simulink model "uz_mpc_6ph"  (R2024b)
settings: Solver=FixedStepDiscrete  StartTime=0.0  StopTime=0.003  RelTol=1e-3
values from neighbouring files (symbols this model uses):
  IB = sqrt(2)*IR    [uz_mpc_6ph_init.m]    (also in uz_mpc_6ph_state_machine_init.m)
  id_ref = 0.0    (= 0)    [uz_mpc_6ph_init.m]    (also in uz_mpc_6ph_state_machine_init.m)
  iq_ref = 15.0    (= 15)    [uz_mpc_6ph_init.m]    (also in uz_mpc_6ph_state_machine_init.m = 3)
  ix_ref = 0.0    (= 0)    [uz_mpc_6ph_init.m]    (also in uz_mpc_6ph_state_machine_init.m)
  iy_ref = 0.0    (= 0)    [uz_mpc_6ph_init.m]    (also in uz_mpc_6ph_state_machine_init.m)
  lambda_d = 1.0    (= 1)    [uz_mpc_6ph_init.m]    (also in uz_mpc_6ph_state_machine_init.m)
  lambda_q = 1.0    (= 1)    [uz_mpc_6ph_init.m]    (also in uz_mpc_6ph_state_machine_init.m)
  lambda_u = 0.0    (= 0)    [uz_mpc_6ph_init.m]    (also in uz_mpc_6ph_state_machine_init.m)
  lambda_x = 1.0    (= 1)    [uz_mpc_6ph_init.m]    (also in uz_mpc_6ph_state_machine_init.m)
  lambda_y = 1.0    (= 1)    [uz_mpc_6ph_init.m]    (also in uz_mpc_6ph_state_machine_init.m)
  Ld_over_LB = Ld/LB    [uz_mpc_6ph_init.m]    (also in uz_mpc_6ph_state_machine_init.m)
  Lq_over_LB = Lq/LB    [uz_mpc_6ph_init.m]    (also in uz_mpc_6ph_state_machine_init.m)
  n_rpm = 2200.0    (= 2200)    [uz_mpc_6ph_init.m]    (also in uz_mpc_6ph_state_machine_init.m = 1200)
  omegaB = nR*2*pi()/60*p    [uz_mpc_6ph_init.m]    (also in uz_mpc_6ph_state_machine_init.m)
  p = 5    [uz_mpc_6ph_init.m]    (also in uz_mpc_6ph_state_machine_init.m)
  psi_pm_over_psiB = psi_pm/psiB    [uz_mpc_6ph_init.m]    (also in uz_mpc_6ph_state_machine_init.m)
  Rs_over_ZB = Rs/ZB    [uz_mpc_6ph_init.m]    (also in uz_mpc_6ph_state_machine_init.m)
  t_ADC = 1/f_ADC    (= 1e-05)    [uz_mpc_6ph_init.m]    (also in uz_mpc_6ph_state_machine_init.m)
  t_clock = 1/f_clock    (= 1e-08)    [uz_mpc_6ph_init.m]    (also in uz_mpc_6ph_state_machine_init.m)
  Ts_times_ZB_over_Ld = Ts*ZB/Ld    [uz_mpc_6ph_init.m]    (also in uz_mpc_6ph_state_machine_init.m)
  Ts_times_ZB_over_Lq = Ts*ZB/Lq    [uz_mpc_6ph_init.m]    (also in uz_mpc_6ph_state_machine_init.m)
  Ts_times_ZB_over_Lx = Ts*ZB/Lx    [uz_mpc_6ph_init.m]    (also in uz_mpc_6ph_state_machine_init.m)
  Ts_times_ZB_over_Ly = Ts*ZB/Ly    [uz_mpc_6ph_init.m]    (also in uz_mpc_6ph_state_machine_init.m)
  v_dc = 565.0    (= 565)    [uz_mpc_6ph_init.m]    (also in uz_mpc_6ph_state_machine_init.m)
  VB = sqrt(2/3)*VR    [uz_mpc_6ph_init.m]    (also in uz_mpc_6ph_state_machine_init.m)
libraries: nesl_utility x32, fl_lib x29, simulink x23, ee_lib x12, hdlsllib x2, spsAlphaBetaZerotodq0Lib x1, batteryecm_lib x1
(part 3 of 4)

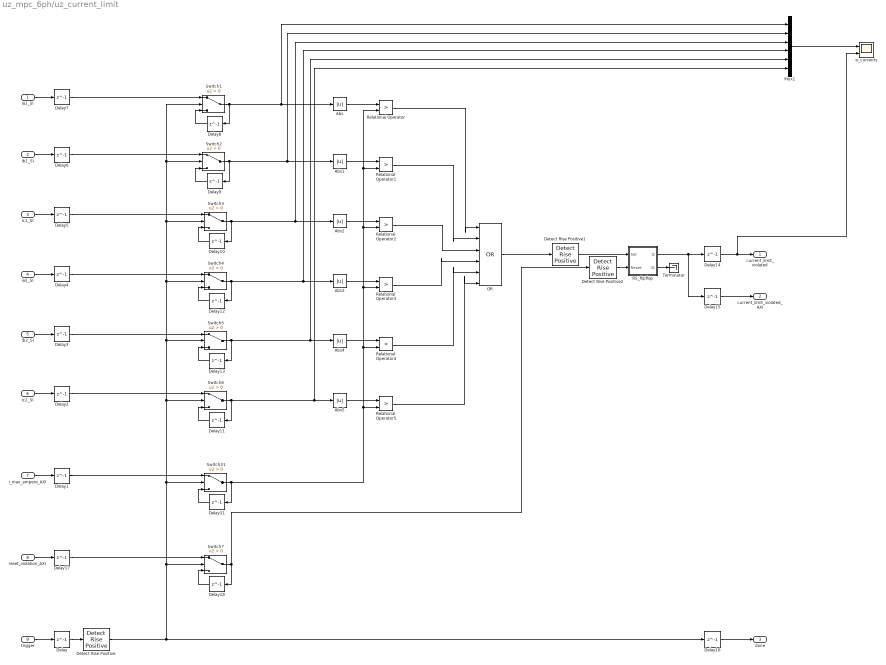
== system uz_mpc_6ph/uz_current_limit ==
  ia1_SI : Inport
  ib1_SI : Inport  Port=2
  ic1_SI : Inport  Port=3
  ia2_SI : Inport  Port=4
  ib2_SI : Inport  Port=5
  ic2_SI : Inport  Port=6
  i_max_ampere_AXI : Inport  Port=7
  reset_violation_AXI : Inport  Port=8
  trigger : Inport  Port=9
  Abs{,1..5} (6 alike) : Abs  SaturateOnIntegerOverflow=off
  Delay{,2..16} (16 alike) : Delay  DelayLength=1
  Delay{1,17..18,31} (4 alike) : Delay  DelayLength=1  InitialCondition=0
  Detect Rise Positive : simulink/Logic and Bit Operations/Detect Rise Positive  vinit=0  OutDataTypeStr=boolean
  Detect Rise Positive1 : simulink/Logic and Bit Operations/Detect Rise Positive  vinit=0  OutDataTypeStr=boolean
  Detect Rise Positive2 : simulink/Logic and Bit Operations/Detect Rise Positive  vinit=0  OutDataTypeStr=boolean
  Mux1 : Mux  Inputs=6
  OR : Logic  Operator=OR  Inputs=6  IconShape=distinctive  AllPortsSameDT=off  OutDataTypeStr=boolean
  RS_flipflop : Subsystem
  Relational Operator{,1..5} (6 alike) : RelationalOperator  Operator=>  OutDataTypeStr=boolean  RndMeth=Simplest  InputSameDT=off
  Switch{1..7,31} (8 alike) : Switch  Criteria=u2 > Threshold  SaturateOnIntegerOverflow=off  InputSameDT=off
  Terminator : Terminator
  si_currents : Scope  NumInputPorts=2
  current_limit_violated : Outport  VectorParamsAs1DForOutWhenUnconnected=off
  current_limit_violated_AXI : Outport  Port=2  VectorParamsAs1DForOutWhenUnconnected=off
  done : Outport  Port=3  VectorParamsAs1DForOutWhenUnconnected=off
  wires:
  Abs/1 -> Relational Operator/1
  Abs1/1 -> Relational Operator1/1
  Abs2/1 -> Relational Operator2/1
  Abs3/1 -> Relational Operator3/1
  Abs4/1 -> Relational Operator4/1
  Abs5/1 -> Relational Operator5/1
  Switch31/1 -> Relational Operator5/2, Relational Operator4/2, Relational Operator3/2, Relational Operator2/2, Relational Operator1/2, Relational Operator/2, Delay31/1
  trigger/1 -> Delay/1
  Delay/1 -> Detect Rise Positive/1
  Delay31/1 -> Switch31/3
  i_max_ampere_AXI/1 -> Delay1/1
  Delay1/1 -> Switch31/1
  ia1_SI/1 -> Delay7/1
  ib1_SI/1 -> Delay6/1
  ic1_SI/1 -> Delay5/1
  ia2_SI/1 -> Delay4/1
  ib2_SI/1 -> Delay3/1
  ic2_SI/1 -> Delay2/1
  Delay7/1 -> Switch1/1
  Delay6/1 -> Switch2/1
  Delay5/1 -> Switch3/1
  Delay4/1 -> Switch4/1
  Delay3/1 -> Switch5/1
  Delay2/1 -> Switch6/1
  Detect Rise Positive/1 -> Switch7/2, Switch6/2, Switch5/2, Switch4/2, Switch3/2, Switch2/2, Switch1/2, Switch31/2, Delay16/1
  Delay11/1 -> Switch6/3
  Delay13/1 -> Switch5/3
  Delay12/1 -> Switch4/3
  Delay10/1 -> Switch3/3
  Delay9/1 -> Switch2/3
  Delay8/1 -> Switch1/3
  Switch1/1 -> Mux1/1, Abs/1, Delay8/1
  Switch2/1 -> Delay9/1, Mux1/2, Abs1/1
  Switch3/1 -> Delay10/1, Mux1/3, Abs2/1
  Switch4/1 -> Delay12/1, Mux1/4, Abs3/1
  Switch5/1 -> Delay13/1, Mux1/5, Abs4/1
  Switch6/1 -> Delay11/1, Mux1/6, Abs5/1
  Relational Operator/1 -> OR/1
  Relational Operator1/1 -> OR/2
  Relational Operator2/1 -> OR/3
  Relational Operator3/1 -> OR/4
  Relational Operator5/1 -> OR/6
  OR/1 -> Detect Rise Positive1/1
  Delay16/1 -> done/1
  Delay15/1 -> current_limit_violated_AXI/1
  Relational Operator4/1 -> OR/5
  Mux1/1 -> si_currents/1
  Delay14/1 -> si_currents/2, current_limit_violated/1
  RS_flipflop/1(Q) -> Delay15/1, Delay14/1
  RS_flipflop/2(!Q) -> Terminator/1
  reset_violation_AXI/1 -> Delay17/1
  Delay18/1 -> Switch7/3
  Switch7/1 -> Delay18/1, Detect Rise Positive2/1
  Delay17/1 -> Switch7/1
  Detect Rise Positive1/1 -> RS_flipflop/1(Set)
  Detect Rise Positive2/1 -> RS_flipflop/2(Reset)

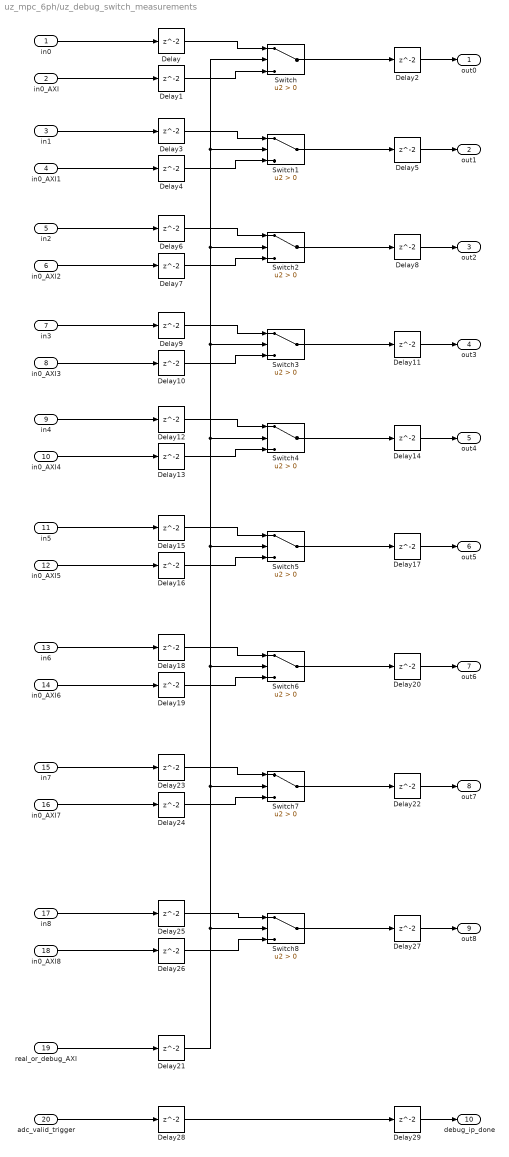
== system uz_mpc_6ph/uz_debug_switch_measurements ==
  in0 : Inport
  in0_AXI : Inport  Port=2
  in1 : Inport  Port=3
  in0_AXI1 : Inport  Port=4
  in2 : Inport  Port=5
  in0_AXI2 : Inport  Port=6
  in3 : Inport  Port=7
  in0_AXI3 : Inport  Port=8
  in4 : Inport  Port=9
  in0_AXI4 : Inport  Port=10
  in5 : Inport  Port=11
  in0_AXI5 : Inport  Port=12
  in6 : Inport  Port=13
  in0_AXI6 : Inport  Port=14
  in7 : Inport  Port=15
  in0_AXI7 : Inport  Port=16
  in8 : Inport  Port=17
  in0_AXI8 : Inport  Port=18
  real_or_debug_AXI : Inport  Port=19
  adc_valid_trigger : Inport  Port=20
  Delay{,1..29} (30 alike) : Delay
  Switch{,1..8} (9 alike) : Switch  Criteria=u2 > Threshold  SaturateOnIntegerOverflow=off  InputSameDT=off
  out0 : Outport  VectorParamsAs1DForOutWhenUnconnected=off
  out1 : Outport  Port=2  VectorParamsAs1DForOutWhenUnconnected=off
  out2 : Outport  Port=3  VectorParamsAs1DForOutWhenUnconnected=off
  out3 : Outport  Port=4  VectorParamsAs1DForOutWhenUnconnected=off
  out4 : Outport  Port=5  VectorParamsAs1DForOutWhenUnconnected=off
  out5 : Outport  Port=6  VectorParamsAs1DForOutWhenUnconnected=off
  out6 : Outport  Port=7  VectorParamsAs1DForOutWhenUnconnected=off
  out7 : Outport  Port=8  VectorParamsAs1DForOutWhenUnconnected=off
  out8 : Outport  Port=9  VectorParamsAs1DForOutWhenUnconnected=off
  debug_ip_done : Outport  Port=10  VectorParamsAs1DForOutWhenUnconnected=off
  wires:
  in0/1 -> Delay/1
  in0_AXI/1 -> Delay1/1
  Delay/1 -> Switch/1
  Delay1/1 -> Switch/3
  Switch/1 -> Delay2/1
  Delay2/1 -> out0/1
  in0_AXI1/1 -> Delay4/1
  Delay5/1 -> out1/1
  in1/1 -> Delay3/1
  Delay4/1 -> Switch1/3
  Delay3/1 -> Switch1/1
  Switch1/1 -> Delay5/1
  in0_AXI2/1 -> Delay7/1
  Delay8/1 -> out2/1
  in2/1 -> Delay6/1
  Delay7/1 -> Switch2/3
  Delay6/1 -> Switch2/1
  Switch2/1 -> Delay8/1
  in0_AXI3/1 -> Delay10/1
  Delay11/1 -> out3/1
  in3/1 -> Delay9/1
  Delay10/1 -> Switch3/3
  Delay9/1 -> Switch3/1
  Switch3/1 -> Delay11/1
  in0_AXI4/1 -> Delay13/1
  Delay14/1 -> out4/1
  in4/1 -> Delay12/1
  Delay13/1 -> Switch4/3
  Delay12/1 -> Switch4/1
  Switch4/1 -> Delay14/1
  in0_AXI5/1 -> Delay16/1
  Delay17/1 -> out5/1
  in5/1 -> Delay15/1
  Delay16/1 -> Switch5/3
  Delay15/1 -> Switch5/1
  Switch5/1 -> Delay17/1
  in0_AXI6/1 -> Delay19/1
  Delay20/1 -> out6/1
  in6/1 -> Delay18/1
  Delay19/1 -> Switch6/3
  Delay18/1 -> Switch6/1
  Switch6/1 -> Delay20/1
  real_or_debug_AXI/1 -> Delay21/1
  Delay22/1 -> out7/1
  Delay23/1 -> Switch7/1
  Delay24/1 -> Switch7/3
  Switch7/1 -> Delay22/1
  in0_AXI7/1 -> Delay24/1
  in7/1 -> Delay23/1
  in0_AXI8/1 -> Delay26/1
  in8/1 -> Delay25/1
  Delay27/1 -> out8/1
  Switch8/1 -> Delay27/1
  Delay25/1 -> Switch8/1
  Delay26/1 -> Switch8/3
  Delay21/1 -> Switch/2, Switch1/2, Switch2/2, Switch3/2, Switch4/2, Switch5/2, Switch6/2, Switch7/2, Switch8/2
  Delay28/1 -> Delay29/1
  Delay29/1 -> debug_ip_done/1
  adc_valid_trigger/1 -> Delay28/1

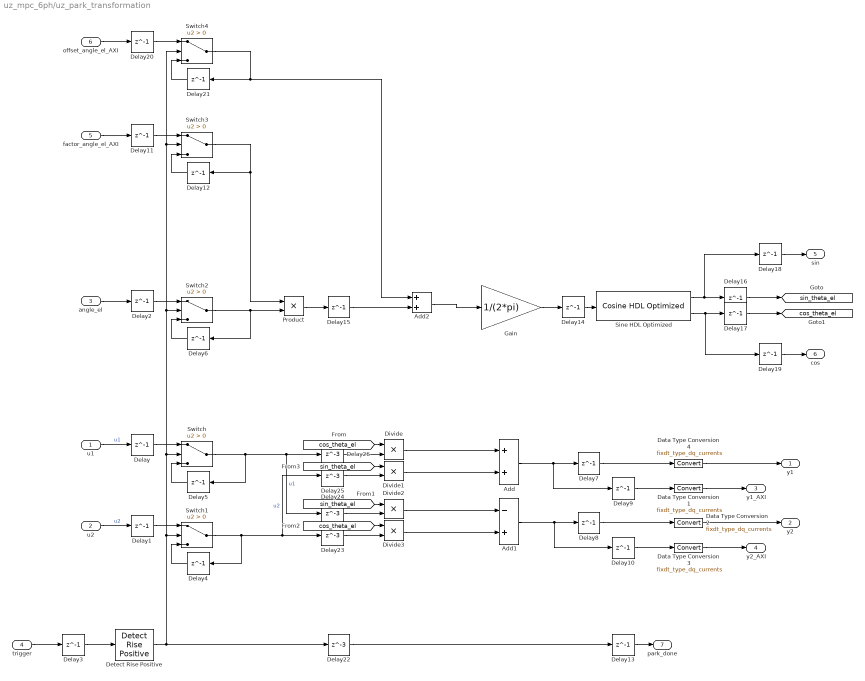
== system uz_mpc_6ph/uz_park_transformation ==
  u1 : Inport
  u2 : Inport  Port=2
  angle_el : Inport  Port=3
  trigger : Inport  Port=4
  factor_angle_el_AXI : Inport  Port=5
  offset_angle_el_AXI : Inport  Port=6
  Add : Sum  OutDataTypeStr=fixdt(1,27,16)
  Add1 : Sum  Inputs=-+  OutDataTypeStr=fixdt(1,27,16)
  Add2 : Sum  AccumDataTypeStr=fixdt(1,27,20)
  Data Type Conversion{1..4} (4 alike) : DataTypeConversion  OutDataTypeStr=fixdt_type_dq_currents  SaturateOnIntegerOverflow=off  RndMeth=Floor
  Delay{,1..21} (22 alike) : Delay  DelayLength=1
  Delay{22..26} (5 alike) : Delay  DelayLength=3
  Detect Rise Positive : simulink/Logic and Bit Operations/Detect Rise Positive  vinit=0  OutDataTypeStr=boolean
  Divide{,1..3} (4 alike) : Product  Inputs=**  OutDataTypeStr=fixdt(1,27,16)
  Gain : Gain  Gain=1/(2*pi)  OutDataTypeStr=fixdt(1,27,20)
  Product : Product  OutDataTypeStr=fixdt(1,27,20)
  Sine HDL Optimized : hdlsllib/Lookup Tables/Cosine HDL Optimized  OutputFormula=sin(2*pi*u) and cos(2*pi*u)  NumDataPoints=256  TableDataTypeStr=fixdt(0,26,20)  SimulateLUTROMDelay=off
  Switch{,1..4} (5 alike) : Switch  Criteria=u2 > Threshold  SaturateOnIntegerOverflow=off  InputSameDT=off
  y1 : Outport  VectorParamsAs1DForOutWhenUnconnected=off
  y2 : Outport  Port=2  VectorParamsAs1DForOutWhenUnconnected=off
  y1_AXI : Outport  Port=3  VectorParamsAs1DForOutWhenUnconnected=off
  y2_AXI : Outport  Port=4  VectorParamsAs1DForOutWhenUnconnected=off
  sin : Outport  Port=5  VectorParamsAs1DForOutWhenUnconnected=off
  cos : Outport  Port=6  VectorParamsAs1DForOutWhenUnconnected=off
  park_done : Outport  Port=7  VectorParamsAs1DForOutWhenUnconnected=off
  tag scope: cos_theta_el=global, sin_theta_el=global
  wires:
  Switch1/1 -> Delay4/1, Delay25/1, Delay23/1  "u2"
  Divide2/1 -> Add1/1
  Divide3/1 -> Add1/2
  [cos_theta_el] -> Divide3/1
  Switch/1 -> Delay24/1, Delay26/1, Delay5/1  "u1"
  [sin_theta_el] -> Divide2/1
  Divide1/1 -> Add/2
  [cos_theta_el] -> Divide/1
  [sin_theta_el] -> Divide1/1
  Add/1 -> Delay9/1, Delay7/1
  Add1/1 -> Delay10/1, Delay8/1
  Divide/1 -> Add/1
  angle_el/1 -> Delay2/1
  Sine HDL Optimized/2 -> Delay19/1, Delay17/1
  Sine HDL Optimized/1 -> Delay18/1, Delay16/1
  Gain/1 -> Delay14/1
  u1/1 -> Delay/1  "u1"
  u2/1 -> Delay1/1  "u2"
  Delay/1 -> Switch/1
  Delay1/1 -> Switch1/1
  Delay2/1 -> Switch2/1
  trigger/1 -> Delay3/1
  Delay4/1 -> Switch1/3
  Delay5/1 -> Switch/3
  Delay6/1 -> Switch2/3
  Delay7/1 -> Data Type Conversion4/1
  Switch2/1 -> Product/2, Delay6/1
  Switch3/1 -> Product/1, Delay12/1
  factor_angle_el_AXI/1 -> Delay11/1
  Delay12/1 -> Switch3/3
  Delay11/1 -> Switch3/1
  Product/1 -> Delay15/1
  Delay3/1 -> Detect Rise Positive/1
  Delay13/1 -> park_done/1
  Delay14/1 -> Sine HDL Optimized/1
  Delay16/1 -> [sin_theta_el]
  Delay17/1 -> [cos_theta_el]
  Delay18/1 -> sin/1
  Delay19/1 -> cos/1
  Add2/1 -> Gain/1
  Delay20/1 -> Switch4/1
  Switch4/1 -> Add2/1, Delay21/1
  Detect Rise Positive/1 -> Delay22/1, Switch1/2, Switch/2, Switch4/2, Switch3/2, Switch2/2
  Delay21/1 -> Switch4/3
  offset_angle_el_AXI/1 -> Delay20/1
  Delay15/1 -> Add2/2
  Delay22/1 -> Delay13/1
  Delay23/1 -> Divide3/2
  Delay24/1 -> Divide2/2
  Delay25/1 -> Divide1/2
  Delay26/1 -> Divide/2
  Data Type Conversion4/1 -> y1/1
  Delay9/1 -> Data Type Conversion1/1
  Delay8/1 -> Data Type Conversion2/1
  Delay10/1 -> Data Type Conversion3/1
  Data Type Conversion1/1 -> y1_AXI/1
  Data Type Conversion2/1 -> y2/1
  Data Type Conversion3/1 -> y2_AXI/1

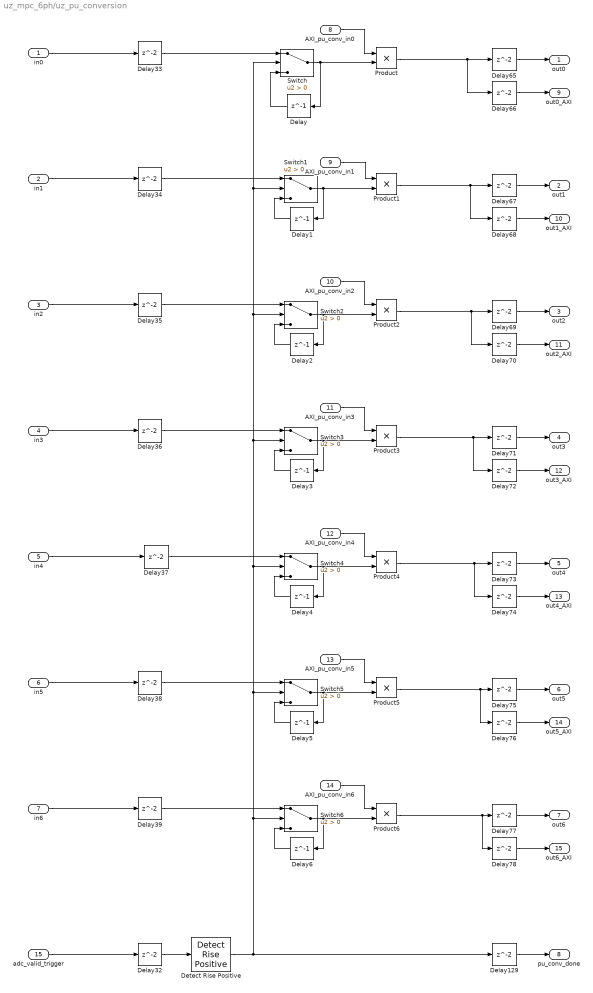
== system uz_mpc_6ph/uz_pu_conversion ==
  in0 : Inport  OutDataTypeStr=fixdt(1,27,15)
  in1 : Inport  Port=2  OutDataTypeStr=fixdt(1,27,15)
  in2 : Inport  Port=3  OutDataTypeStr=fixdt(1,27,15)
  in3 : Inport  Port=4  OutDataTypeStr=fixdt(1,27,15)
  in4 : Inport  Port=5  OutDataTypeStr=fixdt(1,27,15)
  in5 : Inport  Port=6  OutDataTypeStr=fixdt(1,27,15)
  in6 : Inport  Port=7  OutDataTypeStr=fixdt(1,27,15)
  AXI_pu_conv_in0 : Inport  Port=8  OutDataTypeStr=fixdt(0,18,18)
  AXI_pu_conv_in1 : Inport  Port=9  OutDataTypeStr=fixdt(0,18,18)
  AXI_pu_conv_in2 : Inport  Port=10  OutDataTypeStr=fixdt(0,18,18)
  AXI_pu_conv_in3 : Inport  Port=11  OutDataTypeStr=fixdt(0,18,18)
  AXI_pu_conv_in4 : Inport  Port=12  OutDataTypeStr=fixdt(0,18,18)
  AXI_pu_conv_in5 : Inport  Port=13  OutDataTypeStr=fixdt(0,18,18)
  AXI_pu_conv_in6 : Inport  Port=14  OutDataTypeStr=fixdt(0,18,18)
  adc_valid_trigger : Inport  Port=15  OutDataTypeStr=boolean
  Delay{,1..6} (7 alike) : Delay  DelayLength=1
  Delay{32..39,65..78,129} (23 alike) : Delay
  Detect Rise Positive : simulink/Logic and Bit Operations/Detect Rise Positive  vinit=0  OutDataTypeStr=boolean
  Product{,1..6} (7 alike) : Product  OutDataTypeStr=pu_fixdt_type
  Switch{,1..6} (7 alike) : Switch  Criteria=u2 > Threshold  SaturateOnIntegerOverflow=off  InputSameDT=off
  out0 : Outport
  out1 : Outport  Port=2
  out2 : Outport  Port=3
  out3 : Outport  Port=4
  out4 : Outport  Port=5
  out5 : Outport  Port=6
  out6 : Outport  Port=7
  pu_conv_done : Outport  Port=8  OutDataTypeStr=boolean  LockScale=on
  out0_AXI : Outport  Port=9
  out1_AXI : Outport  Port=10
  out2_AXI : Outport  Port=11
  out3_AXI : Outport  Port=12
  out4_AXI : Outport  Port=13
  out5_AXI : Outport  Port=14
  out6_AXI : Outport  Port=15
  wires:
  AXI_pu_conv_in0/1 -> Product/1
  Product/1 -> Delay65/1, Delay66/1
  AXI_pu_conv_in1/1 -> Product1/1
  Product1/1 -> Delay67/1, Delay68/1
  AXI_pu_conv_in2/1 -> Product2/1
  Product3/1 -> Delay71/1, Delay72/1
  Product2/1 -> Delay69/1, Delay70/1
  AXI_pu_conv_in3/1 -> Product3/1
  AXI_pu_conv_in4/1 -> Product4/1
  Product6/1 -> Delay77/1, Delay78/1
  Product5/1 -> Delay75/1, Delay76/1
  AXI_pu_conv_in6/1 -> Product6/1
  Product4/1 -> Delay73/1, Delay74/1
  AXI_pu_conv_in5/1 -> Product5/1
  Switch/1 -> Product/2, Delay/1
  Delay/1 -> Switch/3
  Switch1/1 -> Product1/2, Delay1/1
  Delay1/1 -> Switch1/3
  Switch2/1 -> Product2/2, Delay2/1
  Delay2/1 -> Switch2/3
  Switch3/1 -> Product3/2, Delay3/1
  Delay3/1 -> Switch3/3
  Switch4/1 -> Product4/2, Delay4/1
  Delay4/1 -> Switch4/3
  Switch5/1 -> Product5/2, Delay5/1
  Delay5/1 -> Switch5/3
  Switch6/1 -> Product6/2, Delay6/1
  Delay6/1 -> Switch6/3
  Detect Rise Positive/1 -> Delay129/1, Switch6/2, Switch5/2, Switch3/2, Switch2/2, Switch1/2, Switch/2, Switch4/2
  adc_valid_trigger/1 -> Delay32/1
  Delay32/1 -> Detect Rise Positive/1
  in0/1 -> Delay33/1
  Delay33/1 -> Switch/1
  in1/1 -> Delay34/1
  Delay34/1 -> Switch1/1
  in2/1 -> Delay35/1
  Delay35/1 -> Switch2/1
  in3/1 -> Delay36/1
  Delay36/1 -> Switch3/1
  in4/1 -> Delay37/1
  Delay37/1 -> Switch4/1
  in5/1 -> Delay38/1
  Delay38/1 -> Switch5/1
  in6/1 -> Delay39/1
  Delay39/1 -> Switch6/1
  Delay65/1 -> out0/1
  Delay66/1 -> out0_AXI/1
  Delay67/1 -> out1/1
  Delay68/1 -> out1_AXI/1
  Delay69/1 -> out2/1
  Delay70/1 -> out2_AXI/1
  Delay71/1 -> out3/1
  Delay72/1 -> out3_AXI/1
  Delay73/1 -> out4/1
  Delay74/1 -> out4_AXI/1
  Delay75/1 -> out5/1
  Delay76/1 -> out5_AXI/1
  Delay77/1 -> out6/1
  Delay78/1 -> out6_AXI/1
  Delay129/1 -> pu_conv_done/1

== system uz_mpc_6ph/uz_vsd_6ph_30deg ==
  a1 : Inport
  b1 : Inport  Port=2
  c1 : Inport  Port=3
  a2 : Inport  Port=4
  b2 : Inport  Port=5
  c2 : Inport  Port=6
  pu_conv_valid : Inport  Port=7
  Delay{,1..5} (6 alike) : Delay  DelayLength=1
  Delay{6..25} (20 alike) : Delay
  Detect Rise Positive : simulink/Logic and Bit Operations/Detect Rise Positive  vinit=0  OutDataTypeStr=boolean
  Switch{,1..5} (6 alike) : Switch  Criteria=u2 > Threshold  OutDataTypeStr=fixdt_type_vsd  SaturateOnIntegerOverflow=off  InputSameDT=off
  VSD_6ph_30deg : MATLAB Function  TreatAsAtomicUnit=on
  alpha : Outport  OutDataTypeStr=fixdt(1,18,11)  VectorParamsAs1DForOutWhenUnconnected=off
  beta : Outport  Port=2  OutDataTypeStr=fixdt(1,18,11)  VectorParamsAs1DForOutWhenUnconnected=off
  x1 : Outport  Port=3  OutDataTypeStr=fixdt(1,18,11)  VectorParamsAs1DForOutWhenUnconnected=off
  y1 : Outport  Port=4  OutDataTypeStr=fixdt(1,18,11)  VectorParamsAs1DForOutWhenUnconnected=off
  z1 : Outport  Port=5  OutDataTypeStr=fixdt(1,18,11)  VectorParamsAs1DForOutWhenUnconnected=off
  z2 : Outport  Port=6  OutDataTypeStr=fixdt(1,18,11)  VectorParamsAs1DForOutWhenUnconnected=off
  vsd_done : Outport  Port=7  VectorParamsAs1DForOutWhenUnconnected=off
  alpha_AXI : Outport  Port=8  OutDataTypeStr=fixdt(1,18,11)  VectorParamsAs1DForOutWhenUnconnected=off
  beta_AXI : Outport  Port=9  OutDataTypeStr=fixdt(1,18,11)  VectorParamsAs1DForOutWhenUnconnected=off
  x_AXI : Outport  Port=10  OutDataTypeStr=fixdt(1,18,11)  VectorParamsAs1DForOutWhenUnconnected=off
  y_AXI : Outport  Port=11  OutDataTypeStr=fixdt(1,18,11)  VectorParamsAs1DForOutWhenUnconnected=off
  z1_AXI : Outport  Port=12  OutDataTypeStr=fixdt(1,18,11)  VectorParamsAs1DForOutWhenUnconnected=off
  z2_AXI : Outport  Port=13  OutDataTypeStr=fixdt(1,18,11)  VectorParamsAs1DForOutWhenUnconnected=off
  wires:
  VSD_6ph_30deg/1(alpha) -> Delay20/1, Delay14/1
  VSD_6ph_30deg/2(beta) -> Delay21/1, Delay15/1
  VSD_6ph_30deg/3(x1) -> Delay22/1, Delay16/1
  VSD_6ph_30deg/4(y1) -> Delay23/1, Delay17/1
  VSD_6ph_30deg/5(z1) -> Delay24/1, Delay18/1
  VSD_6ph_30deg/6(z2) -> Delay25/1, Delay19/1
  pu_conv_valid/1 -> Delay6/1
  Detect Rise Positive/1 -> Switch5/2, Switch4/2, Switch3/2, Switch2/2, Switch1/2, Switch/2, Delay13/1
  Delay/1 -> Switch/3
  Switch/1 -> VSD_6ph_30deg/1(a1), Delay/1
  Delay1/1 -> Switch1/3
  Switch1/1 -> VSD_6ph_30deg/2(b1), Delay1/1
  Delay2/1 -> Switch2/3
  Switch2/1 -> VSD_6ph_30deg/3(c1), Delay2/1
  Delay3/1 -> Switch3/3
  Switch3/1 -> VSD_6ph_30deg/4(a2), Delay3/1
  Delay4/1 -> Switch4/3
  Switch4/1 -> VSD_6ph_30deg/5(b2), Delay4/1
  Delay5/1 -> Switch5/3
  Switch5/1 -> VSD_6ph_30deg/6(c2), Delay5/1
  a1/1 -> Delay7/1
  b1/1 -> Delay8/1
  c1/1 -> Delay9/1
  a2/1 -> Delay10/1
  b2/1 -> Delay11/1
  c2/1 -> Delay12/1
  Delay6/1 -> Detect Rise Positive/1
  Delay7/1 -> Switch/1
  Delay8/1 -> Switch1/1
  Delay9/1 -> Switch2/1
  Delay10/1 -> Switch3/1
  Delay11/1 -> Switch4/1
  Delay12/1 -> Switch5/1
  Delay13/1 -> vsd_done/1
  Delay14/1 -> alpha/1
  Delay15/1 -> beta/1
  Delay16/1 -> x1/1
  Delay17/1 -> y1/1
  Delay18/1 -> z1/1
  Delay19/1 -> z2/1
  Delay20/1 -> alpha_AXI/1
  Delay21/1 -> beta_AXI/1
  Delay22/1 -> x_AXI/1
  Delay23/1 -> y_AXI/1
  Delay24/1 -> z1_AXI/1
  Delay25/1 -> z2_AXI/1

== system uz_mpc_6ph/ctrl_state_machine/Subsystem ==
  Set : Inport
  Reset : Inport  Port=2
  Constant1 : Constant  Value=0  OutDataTypeStr=uint32  SampleTime=-1
  Data Type Conversion1 : DataTypeConversion  OutDataTypeStr=boolean  SaturateOnIntegerOverflow=off  RndMeth=Floor
  Data Type Conversion2 : DataTypeConversion  OutDataTypeStr=boolean  SaturateOnIntegerOverflow=off  RndMeth=Floor
  Logical Operator : Logic  Operator=NOT  AllPortsSameDT=off  OutDataTypeStr=boolean
  Logical Operator1 : Logic  AllPortsSameDT=off  OutDataTypeStr=boolean
  Logical Operator2 : Logic  Operator=OR  AllPortsSameDT=off  OutDataTypeStr=boolean
  Logical Operator3 : Logic  Operator=NOT  AllPortsSameDT=off  OutDataTypeStr=boolean
  Logical Operator4 : Logic  Operator=OR  AllPortsSameDT=off  OutDataTypeStr=boolean
  Logical Operator5 : Logic  AllPortsSameDT=off  OutDataTypeStr=boolean
  Switch1 : Switch  Criteria=u2 > Threshold  Threshold=1  SaturateOnIntegerOverflow=off  InputSameDT=off
  Unit Delay : UnitDelay  InitialCondition=1  SampleTime=t_clock  HasFrameUpgradeWarning=on
  Q : Outport  VectorParamsAs1DForOutWhenUnconnected=off
  !Q : Outport  Port=2  VectorParamsAs1DForOutWhenUnconnected=off
  wires:
  Logical Operator/1 -> Logical Operator1/2, Logical Operator5/1
  Reset/1 -> Data Type Conversion2/1
  Constant1/1 -> Switch1/2
  Logical Operator4/1 -> Switch1/1
  Data Type Conversion1/1 -> Logical Operator2/1, Logical Operator4/1
  Switch1/1 -> Q/1, Unit Delay/1, Logical Operator3/1
  Logical Operator3/1 -> !Q/1
  Set/1 -> Data Type Conversion1/1
  Logical Operator2/1 -> Logical Operator1/1
  Unit Delay/1 -> Logical Operator2/2, Logical Operator5/2
  Logical Operator5/1 -> Logical Operator4/2
  Logical Operator1/1 -> Switch1/3
  Data Type Conversion2/1 -> Logical Operator/1

== system uz_mpc_6ph/ctrl_state_machine/Subsystem2 ==
  Set : Inport
  Reset : Inport  Port=2
  Constant1 : Constant  Value=0  OutDataTypeStr=uint32  SampleTime=-1
  Data Type Conversion1 : DataTypeConversion  OutDataTypeStr=boolean  SaturateOnIntegerOverflow=off  RndMeth=Floor
  Data Type Conversion2 : DataTypeConversion  OutDataTypeStr=boolean  SaturateOnIntegerOverflow=off  RndMeth=Floor
  Logical Operator : Logic  Operator=NOT  AllPortsSameDT=off  OutDataTypeStr=boolean
  Logical Operator1 : Logic  AllPortsSameDT=off  OutDataTypeStr=boolean
  Logical Operator2 : Logic  Operator=OR  AllPortsSameDT=off  OutDataTypeStr=boolean
  Logical Operator3 : Logic  Operator=NOT  AllPortsSameDT=off  OutDataTypeStr=boolean
  Logical Operator4 : Logic  Operator=OR  AllPortsSameDT=off  OutDataTypeStr=boolean
  Logical Operator5 : Logic  AllPortsSameDT=off  OutDataTypeStr=boolean
  Switch1 : Switch  Criteria=u2 > Threshold  Threshold=1  SaturateOnIntegerOverflow=off  InputSameDT=off
  Unit Delay : UnitDelay  SampleTime=t_clock  HasFrameUpgradeWarning=on
  Q : Outport  VectorParamsAs1DForOutWhenUnconnected=off
  !Q : Outport  Port=2  VectorParamsAs1DForOutWhenUnconnected=off
  wires:
  Logical Operator/1 -> Logical Operator1/2, Logical Operator5/1
  Reset/1 -> Data Type Conversion2/1
  Constant1/1 -> Switch1/2
  Logical Operator4/1 -> Switch1/1
  Data Type Conversion1/1 -> Logical Operator2/1, Logical Operator4/1
  Switch1/1 -> Q/1, Unit Delay/1, Logical Operator3/1
  Logical Operator3/1 -> !Q/1
  Set/1 -> Data Type Conversion1/1
  Logical Operator2/1 -> Logical Operator1/1
  Unit Delay/1 -> Logical Operator2/2, Logical Operator5/2
  Logical Operator5/1 -> Logical Operator4/2
  Logical Operator1/1 -> Switch1/3
  Data Type Conversion2/1 -> Logical Operator/1

== system uz_mpc_6ph/ctrl_state_machine/Subsystem4 ==
  Set : Inport
  Reset : Inport  Port=2
  Constant1 : Constant  Value=0  OutDataTypeStr=uint32  SampleTime=-1
  Data Type Conversion1 : DataTypeConversion  OutDataTypeStr=boolean  SaturateOnIntegerOverflow=off  RndMeth=Floor
  Data Type Conversion2 : DataTypeConversion  OutDataTypeStr=boolean  SaturateOnIntegerOverflow=off  RndMeth=Floor
  Logical Operator : Logic  Operator=NOT  AllPortsSameDT=off  OutDataTypeStr=boolean
  Logical Operator1 : Logic  AllPortsSameDT=off  OutDataTypeStr=boolean
  Logical Operator2 : Logic  Operator=OR  AllPortsSameDT=off  OutDataTypeStr=boolean
  Logical Operator3 : Logic  Operator=NOT  AllPortsSameDT=off  OutDataTypeStr=boolean
  Logical Operator4 : Logic  Operator=OR  AllPortsSameDT=off  OutDataTypeStr=boolean
  Logical Operator5 : Logic  AllPortsSameDT=off  OutDataTypeStr=boolean
  Switch1 : Switch  Criteria=u2 > Threshold  Threshold=1  SaturateOnIntegerOverflow=off  InputSameDT=off
  Unit Delay : UnitDelay  SampleTime=t_clock  HasFrameUpgradeWarning=on
  Q : Outport  VectorParamsAs1DForOutWhenUnconnected=off
  !Q : Outport  Port=2  VectorParamsAs1DForOutWhenUnconnected=off
  wires:
  Logical Operator/1 -> Logical Operator1/2, Logical Operator5/1
  Reset/1 -> Data Type Conversion2/1
  Constant1/1 -> Switch1/2
  Logical Operator4/1 -> Switch1/1
  Data Type Conversion1/1 -> Logical Operator2/1, Logical Operator4/1
  Switch1/1 -> Q/1, Unit Delay/1, Logical Operator3/1
  Logical Operator3/1 -> !Q/1
  Set/1 -> Data Type Conversion1/1
  Logical Operator2/1 -> Logical Operator1/1
  Unit Delay/1 -> Logical Operator2/2, Logical Operator5/2
  Logical Operator5/1 -> Logical Operator4/2
  Logical Operator1/1 -> Switch1/3
  Data Type Conversion2/1 -> Logical Operator/1

== system uz_mpc_6ph/ctrl_state_machine/Subsystem7 ==
  Set : Inport
  Reset : Inport  Port=2
  Constant1 : Constant  Value=0  OutDataTypeStr=uint32  SampleTime=-1
  Data Type Conversion1 : DataTypeConversion  OutDataTypeStr=boolean  SaturateOnIntegerOverflow=off  RndMeth=Floor
  Data Type Conversion2 : DataTypeConversion  OutDataTypeStr=boolean  SaturateOnIntegerOverflow=off  RndMeth=Floor
  Logical Operator : Logic  Operator=NOT  AllPortsSameDT=off  OutDataTypeStr=boolean
  Logical Operator1 : Logic  AllPortsSameDT=off  OutDataTypeStr=boolean
  Logical Operator2 : Logic  Operator=OR  AllPortsSameDT=off  OutDataTypeStr=boolean
  Logical Operator3 : Logic  Operator=NOT  AllPortsSameDT=off  OutDataTypeStr=boolean
  Logical Operator4 : Logic  Operator=OR  AllPortsSameDT=off  OutDataTypeStr=boolean
  Logical Operator5 : Logic  AllPortsSameDT=off  OutDataTypeStr=boolean
  Switch1 : Switch  Criteria=u2 > Threshold  Threshold=1  SaturateOnIntegerOverflow=off  InputSameDT=off
  Unit Delay : UnitDelay  InitialCondition=1  SampleTime=t_clock  HasFrameUpgradeWarning=on
  Q : Outport  VectorParamsAs1DForOutWhenUnconnected=off
  !Q : Outport  Port=2  VectorParamsAs1DForOutWhenUnconnected=off
  wires:
  Logical Operator/1 -> Logical Operator1/2, Logical Operator5/1
  Reset/1 -> Data Type Conversion2/1
  Constant1/1 -> Switch1/2
  Logical Operator4/1 -> Switch1/1
  Data Type Conversion1/1 -> Logical Operator2/1, Logical Operator4/1
  Switch1/1 -> Q/1, Unit Delay/1, Logical Operator3/1
  Logical Operator3/1 -> !Q/1
  Set/1 -> Data Type Conversion1/1
  Logical Operator2/1 -> Logical Operator1/1
  Unit Delay/1 -> Logical Operator2/2, Logical Operator5/2
  Logical Operator5/1 -> Logical Operator4/2
  Logical Operator1/1 -> Switch1/3
  Data Type Conversion2/1 -> Logical Operator/1

== system uz_mpc_6ph/ctrl_state_machine/limited_counter ==
  limit : Inport
  enb : Inport  Port=2
  Add : Sum  Inputs=-++  AccumDataTypeStr=uint8
  Constant3 : Constant  Value=0  OutDataTypeStr=uint8  SampleTime=-1
  Constant5 : Constant  OutDataTypeStr=uint8  SampleTime=-1
  Constant6 : Constant  Value=0  OutDataTypeStr=uint8  SampleTime=-1
  Delay4 : Delay  DelayLength=1
  Relational Operator1 : RelationalOperator  OutDataTypeStr=boolean  RndMeth=Simplest  InputSameDT=off
  Switch7 : Switch  Criteria=u2 > Threshold  SaturateOnIntegerOverflow=off  InputSameDT=off
  Switch8 : Switch  Criteria=u2 > Threshold  SaturateOnIntegerOverflow=off  InputSameDT=off
  cnt : Outport
  wires:
  Constant6/1 -> Switch8/3
  Constant3/1 -> Switch7/3
  Switch8/1 -> Add/1  "trigger"
  Delay4/1 -> Add/3, Relational Operator1/1, Switch8/1
  Switch7/1 -> Add/2  "trigger"
  Constant5/1 -> Switch7/1
  Relational Operator1/1 -> Switch8/2
  Add/1 -> cnt/1, Delay4/1
  limit/1 -> Relational Operator1/2
  enb/1 -> Switch7/2

== system uz_mpc_6ph/ctrl_state_machine/resetable_counter ==
  enb : Inport
  rst : Inport  Port=2
  Add : Sum  Inputs=-++  AccumDataTypeStr=uint8
  Add1 : Sum  Inputs=+-  AccumDataTypeStr=uint8
  Constant1 : Constant  Value=0  OutDataTypeStr=uint8  SampleTime=-1
  Constant3 : Constant  Value=0  OutDataTypeStr=uint8  SampleTime=-1
  Constant5 : Constant  OutDataTypeStr=uint8  SampleTime=-1
  Constant6 : Constant  Value=0  OutDataTypeStr=uint8  SampleTime=-1
  Delay4 : Delay  DelayLength=1
  Switch7 : Switch  Criteria=u2 > Threshold  SaturateOnIntegerOverflow=off  InputSameDT=off
  Switch8 : Switch  Criteria=u2 > Threshold  SaturateOnIntegerOverflow=off  InputSameDT=off
  cnt : Outport
  wires:
  Constant6/1 -> Switch8/3
  Constant3/1 -> Switch7/3
  Switch8/1 -> Add/1  "trigger"
  Switch7/1 -> Add/2  "trigger"
  Constant5/1 -> Switch7/1
  Add/1 -> cnt/1, Delay4/1
  enb/1 -> Switch7/2
  Constant1/1 -> Add1/2
  Add1/1 -> Switch8/1
  Delay4/1 -> Add/3, Add1/1
  rst/1 -> Switch8/2

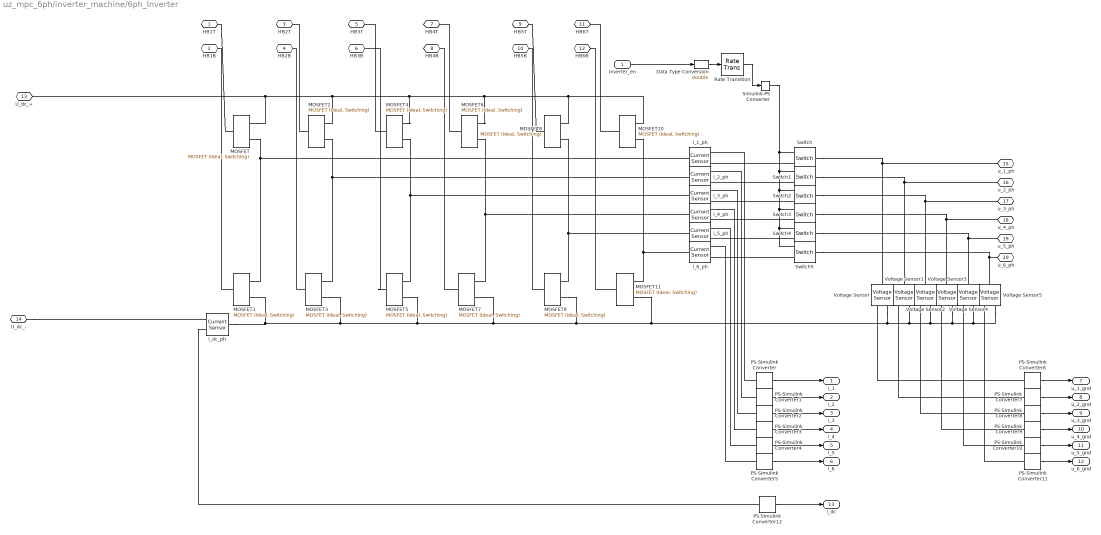
== system uz_mpc_6ph/inverter_machine/6ph_Inverter ==
  inverter_en : Inport  OutDataTypeStr=boolean
  Data Type Conversion : DataTypeConversion  OutDataTypeStr=double  SaturateOnIntegerOverflow=off  RndMeth=Floor
  MOSFET{,1..11} (12 alike) : ee_lib/Semiconductors & Converters/MOSFET (Ideal, Switching)  port_option=ee.enum.controlport.ps  Rds=RDSon Ohm  Goff=1e-6 1/Ohm  Vth=0.7 V  diode_param=2  diode_Vf=diode_fwd_voltage V  diode_Ron=0.001 Ohm  diode_Goff=1e-5 1/Ohm  diode_C=5e-8 F  diode_iRM=-235 A  diode_iF=300 A  diode_idot=-50 A/us  diode_trr_param=1  diode_trr_factor=3  diode_trr=15 us  diode_Qrr=1.5e+3 s*uA  ids_specify=off  ids_priority=None  ids=0 A  ids_nominal_specify=off  ids_nominal_value=1  ids_nominal_unit=A  vds_specify=off  vds_priority=None  vds=0 V  vds_nominal_specify=off  vds_nominal_value=1  vds_nominal_unit=V  vgs_specify=off  vgs_priority=None  vgs=0 V  vgs_nominal_specify=off  vgs_nominal_value=1  vgs_nominal_unit=V  thermal_loss_option=ee.enum.converters.thermalLossOption.constantvalues  Von_data=[0, 1.1, 1.3, 1.45, 1.75, 2.25, 2.7; 0, 1, 1.15, 1.35, 1.7, 2.35, 3] V  Tj=[298.15, 398.15] K  Iout_data=[0, 10, 50, 100, 200, 400, 600] A  Eon_data=[0, .29, 1.43, 2.86, 5.71, 13.14, 22.86; 0, .57, 2.63, 5.14, 10.29, 20.57, 30.29] * 1e-3 J  Eoff_data=[0, .21, 1.07, 2.14, 4.29, 9.86, 17.14; 0, .43, 1.97, 3.86, 7.71, 15.43, 22.71] * 1e-3 J  Eon_data_3D=[zeros(2, 5, 3)] J  Eoff_data_3D=[zeros(2, 5, 3)] J  Tj_loss=[298.15, 448.15] K  Iout_data_loss=[0, 10, 20, 30, 40] A  tabulateWithVds=false  Vds_loss=[0, 150, 300] V  Eon_scalar=22.86e-3 J  Eoff_scalar=17.14e-3 J  Voff=300 V  Iout_scalar=600 A  useCurrentFromPreviousCycle=false  useVoltageFromPreviousCycle=false  diodeModelType=ee.enum.converters.diodeModelType.pwl  diodeTableType=ee.enum.diode.tableType.IfMat  diode_ReverseIVType=ee.enum.diode.diodeReverseIV.constant  diode_IfMat=[.07, .12, .19, 1.75, 4.24, 7.32, 11.2; .16, .3, .72, 2.14, 4.02, 6.35, 9.12] A  diode_VfMat=[.9, 1.15, 1.25, 1.5, 1.75, 2.17, 2.6, 2.85; .58, .68, .75, 1.1, 1.38, 1.77, 2.27, 2.7] V  diode_TjVec=[25, 125] degC  diode_VfVec=[.5, .7, .9, 1.3, 1.7, 2.1, 2.5] V  diode_IfVec=[.1, .2, .5, 1, 2, 4, 7, 10] A  diode_IrMat=[1e-06, 2e-06, 5e-06, 1e-05, 2.5e-05, 5e-05, .0001; 2e-06, 5e-06, 1e-05, 4e-05, 8e-05, .0002, .0005] A  diode_VrMat=[10, 100, 200, 250, 300, 325, 350; 10, 70, 160, 220, 270, 300, 320] V  diode_VrVec=[10, 20, 40, 50, 70, 80, 100] V  diode_IrVec=[1e-06, 2e-06, 5e-06, 1e-05, 2e-05, 5e-05, .0001] A  diode_Vr=-600 V  diode_Ls=150 nH  diode_Erec=0.03 J  diode_rec_loss_model=ee.enum.diode.reverseRecoveryModel.fixed  diode_ErecVal=0 J  diode_scaleWithIandV=true  diode_ErecMat=zeros(2, 3) J  diode_TjrecVec=[298.15, 398.15] K  diode_IfrecVec=[.1, 1, 10] A  diode_IrecVal=10 A  diode_VrecVal=10 V  diode_tFilter=1 / 1000 / 100 s  separateThermalPortForDiode=false  thermal_network_parameterization=ee.enum.thermalNetworkTopology.external  Rth=[.03, .2] K/W  Rth_Cauer=[.03, .1, .2] K/W  Rth_Foster=[.03, .2] K/W  thermal_mass_parameterization=ee.enum.thermalNetwork.timeconstant  thermal_mass=[3, 25] J/K  thermal_mass_Cauer=[3, 10, 25] J/K  thermal_mass_Foster=[33, 50] J/K  thermal_time_constant=[.1, 5] s  thermal_time_constant_Cauer=[.1, 1, 5] s  thermal_time_constant_Foster=[1, 10] s  thermal_mass_initial_temperatures=[25, 25] degC  thermal_mass_initial_temperatures_Cauer=[25, 25, 25] degC  junction_thermal_mass=0.1 J/K  Tvec_initial_Foster=[25, 25, 25, 25] degC  RthDiode=[.03, .2] K/W  RthCauerDiode=[.03, .1, .2] K/W  RthFosterDiode=[.03, .2] K/W  thermalMassDiode=[3, 25] J/K  thermalMassCauerDiode=[3, 10, 25] J/K  thermalMassFosterDiode=[33, 50] J/K  thermalTauDiode=[.1, 5] s  thermalTauCauerDiode=[.1, 1, 5] s  thermalTauFosterDiode=[1, 10] s  thermalMassInitTempDiode=[25, 25] degC  thermalMassInitTempCauerDiode=[25, 25, 25] degC  junctionthermalMassDiode=0.1 J/K  TVecInitialFosterDiode=[25, 25, 25, 25] degC  no_thermal_network=0  mosfet_junction_temperature_specify=off  mosfet_junction_temperature_priority=None  mosfet_junction_temperature=25 degC  mosfet_junction_temperature_nominal_specify=off  mosfet_junction_temperature_nominal_value=1  mosfet_junction_temperature_nominal_unit=degC  diode_junction_temperature_specify=off  diode_junction_temperature_priority=None  diode_junction_temperature=25 degC  diode_junction_temperature_nominal_specify=off  diode_junction_temperature_nominal_value=1  diode_junction_temperature_nominal_unit=degC  Qj_specify=off  Qj_priority=None  Qj=0 W  Qj_nominal_specify=off  Qj_nominal_value=1  Qj_nominal_unit=W  accumulatedSwitchingLosses_specify=off  accumulatedSwitchingLosses_priority=None  accumulatedSwitchingLosses=0 J
  PS-Simulink Converter{,1..5,12} (7 alike) : nesl_utility/PS-Simulink Converter  PhysicalDomain=network_engine_domain  SubClassName=ps_output  LeftPortType=input  RightPortType=output  PseudoPeriodic=off  Frequencies=[]  VectorFormat=1-D array  Unit=A  AffineConversion=off
  PS-Simulink Converter{6..11} (6 alike) : nesl_utility/PS-Simulink Converter  PhysicalDomain=network_engine_domain  SubClassName=ps_output  LeftPortType=input  RightPortType=output  PseudoPeriodic=off  Frequencies=[]  VectorFormat=1-D array  Unit=V  AffineConversion=off
  Rate Transition : RateTransition
  Simulink-PS Converter : nesl_utility/Simulink-PS Converter  PhysicalDomain=network_engine_domain  SubClassName=ps_input  LeftPortType=input  RightPortType=output  PseudoPeriodic=off  Frequencies=[]  NoiseDistribution=none  NoiseParameters=[]  Unit=1  AffineConversion=off  FilteringAndDerivatives=provide  SimscapeFilterOrder=1  InputFilterTimeConstant=0.001  UdotUserProvided=0
  Switch{,1..5} (6 alike) : fl_lib/Electrical/Electrical Elements/Switch  R_closed=0.01 Ohm  G_open=1e-8 1/Ohm  Threshold=0.5  i_specify=off  i_priority=None  i=0 A  i_nominal_specify=off  i_nominal_value=1  i_nominal_unit=A  v_specify=off  v_priority=None  v=0 V  v_nominal_specify=off  v_nominal_value=1  v_nominal_unit=V
  Voltage Sensor{,1..5} (6 alike) : fl_lib/Electrical/Electrical Sensors/Voltage Sensor
  i_1_ph : fl_lib/Electrical/Electrical Sensors/Current Sensor
  i_2_ph : fl_lib/Electrical/Electrical Sensors/Current Sensor
  i_3_ph : fl_lib/Electrical/Electrical Sensors/Current Sensor
  i_4_ph : fl_lib/Electrical/Electrical Sensors/Current Sensor
  i_5_ph : fl_lib/Electrical/Electrical Sensors/Current Sensor
  i_6_ph : fl_lib/Electrical/Electrical Sensors/Current Sensor
  i_dc_ph : fl_lib/Electrical/Electrical Sensors/Current Sensor
  HB1T : PMIOPort  Side=Left
  HB1B : PMIOPort  Port=2  Side=Left
  HB2T : PMIOPort  Port=3  Side=Left
  HB2B : PMIOPort  Port=4  Side=Left
  HB3T : PMIOPort  Port=5  Side=Left
  HB3B : PMIOPort  Port=6  Side=Left
  HB4T : PMIOPort  Port=7  Side=Left
  HB4B : PMIOPort  Port=8  Side=Left
  HB5T : PMIOPort  Port=9  Side=Left
  HB5B : PMIOPort  Port=10  Side=Left
  HB6T : PMIOPort  Port=11  Side=Left
  HB6B : PMIOPort  Port=12  Side=Left
  U_dc_+ : PMIOPort  Port=13  Side=Left
  U_dc_- : PMIOPort  Port=14  Side=Left
  u_1_ph : PMIOPort  Port=15  Side=Right
  u_2_ph : PMIOPort  Port=16  Side=Right
  u_3_ph : PMIOPort  Port=17  Side=Right
  u_4_ph : PMIOPort  Port=18  Side=Right
  u_5_ph : PMIOPort  Port=19  Side=Right
  u_6_ph : PMIOPort  Port=20  Side=Right
  i_1 : Outport  VectorParamsAs1DForOutWhenUnconnected=off
  i_2 : Outport  Port=2  VectorParamsAs1DForOutWhenUnconnected=off
  i_3 : Outport  Port=3  VectorParamsAs1DForOutWhenUnconnected=off
  i_4 : Outport  Port=4  VectorParamsAs1DForOutWhenUnconnected=off
  i_5 : Outport  Port=5  VectorParamsAs1DForOutWhenUnconnected=off
  i_6 : Outport  Port=6  VectorParamsAs1DForOutWhenUnconnected=off
  u_1_gnd : Outport  Port=7  VectorParamsAs1DForOutWhenUnconnected=off
  u_2_gnd : Outport  Port=8  VectorParamsAs1DForOutWhenUnconnected=off
  u_3_gnd : Outport  Port=9  VectorParamsAs1DForOutWhenUnconnected=off
  u_4_gnd : Outport  Port=10  VectorParamsAs1DForOutWhenUnconnected=off
  u_5_gnd : Outport  Port=11  VectorParamsAs1DForOutWhenUnconnected=off
  u_6_gnd : Outport  Port=12  VectorParamsAs1DForOutWhenUnconnected=off
  i_dc : Outport  Port=13  VectorParamsAs1DForOutWhenUnconnected=off
  wires:
  PS-Simulink Converter/1 -> i_1/1
  PS-Simulink Converter1/1 -> i_2/1
  PS-Simulink Converter2/1 -> i_3/1
  PS-Simulink Converter3/1 -> i_4/1
  PS-Simulink Converter4/1 -> i_5/1
  PS-Simulink Converter5/1 -> i_6/1
  PS-Simulink Converter9/1 -> u_4_gnd/1
  PS-Simulink Converter8/1 -> u_3_gnd/1
  PS-Simulink Converter7/1 -> u_2_gnd/1
  PS-Simulink Converter6/1 -> u_1_gnd/1
  PS-Simulink Converter10/1 -> u_5_gnd/1
  PS-Simulink Converter11/1 -> u_6_gnd/1
  PS-Simulink Converter12/1 -> i_dc/1
  inverter_en/1 -> Data Type Conversion/1
  Data Type Conversion/1 -> Rate Transition/1
  Rate Transition/1 -> Simulink-PS Converter/1
  connections:
  MOSFET6/RConn2 -- i_4_ph/LConn1 -- MOSFET7/RConn1
  MOSFET2/RConn2 -- i_2_ph/LConn1 -- MOSFET3/RConn1
  MOSFET4/RConn2 -- i_3_ph/LConn1 -- MOSFET5/RConn1
  MOSFET5/RConn2 -- Voltage Sensor5/RConn2 -- Voltage Sensor4/RConn2 -- Voltage Sensor3/RConn2 -- Voltage Sensor2/RConn2 -- Voltage Sensor1/RConn2 -- Voltage Sensor/RConn2 -- MOSFET11/RConn2 -- MOSFET9/RConn2 -- MOSFET7/RConn2 -- i_dc_ph/LConn1 -- MOSFET1/RConn2 -- MOSFET3/RConn2
  MOSFET/RConn2 -- i_1_ph/LConn1 -- MOSFET1/RConn1
  MOSFET11/LConn1 -- HB6B/RConn1
  MOSFET8/RConn2 -- i_5_ph/LConn1 -- MOSFET9/RConn1
  MOSFET2/LConn1 -- HB2T/RConn1
  MOSFET10/RConn2 -- i_6_ph/LConn1 -- MOSFET11/RConn1
  MOSFET/LConn1 -- HB1T/RConn1
  MOSFET9/LConn1 -- HB5B/RConn1
  MOSFET5/LConn1 -- HB3B/RConn1
  MOSFET1/LConn1 -- HB1B/RConn1
  MOSFET7/LConn1 -- HB4B/RConn1
  MOSFET8/LConn1 -- HB5T/RConn1
  MOSFET4/LConn1 -- HB3T/RConn1
  MOSFET10/LConn1 -- HB6T/RConn1
  MOSFET6/LConn1 -- HB4T/RConn1
  MOSFET3/LConn1 -- HB2B/RConn1
  Voltage Sensor/LConn1 -- Switch/LConn1 -- u_1_ph/RConn1
  Voltage Sensor1/LConn1 -- Switch1/LConn1 -- u_2_ph/RConn1
  Voltage Sensor2/LConn1 -- Switch2/LConn1 -- u_3_ph/RConn1
  Voltage Sensor3/LConn1 -- Switch3/LConn1 -- u_4_ph/RConn1
  Voltage Sensor4/LConn1 -- Switch4/LConn1 -- u_5_ph/RConn1
  Voltage Sensor5/LConn1 -- Switch5/LConn1 -- u_6_ph/RConn1
  PS-Simulink Converter/LConn1 -- i_1_ph/RConn1
  PS-Simulink Converter1/LConn1 -- i_2_ph/RConn1
  PS-Simulink Converter2/LConn1 -- i_3_ph/RConn1
  i_4_ph/RConn1 -- PS-Simulink Converter3/LConn1
  PS-Simulink Converter4/LConn1 -- i_5_ph/RConn1
  PS-Simulink Converter5/LConn1 -- i_6_ph/RConn1
  PS-Simulink Converter6/LConn1 -- Voltage Sensor/RConn1
  PS-Simulink Converter7/LConn1 -- Voltage Sensor1/RConn1
  PS-Simulink Converter8/LConn1 -- Voltage Sensor2/RConn1
  PS-Simulink Converter9/LConn1 -- Voltage Sensor3/RConn1
  PS-Simulink Converter10/LConn1 -- Voltage Sensor4/RConn1
  PS-Simulink Converter11/LConn1 -- Voltage Sensor5/RConn1
  U_dc_-/RConn1 -- i_dc_ph/RConn2
  PS-Simulink Converter12/LConn1 -- i_dc_ph/RConn1
  MOSFET6/RConn1 -- MOSFET/RConn1 -- U_dc_+/RConn1 -- MOSFET2/RConn1 -- MOSFET4/RConn1 -- MOSFET10/RConn1 -- MOSFET8/RConn1
  Switch/RConn2 -- i_1_ph/RConn2
  Switch1/RConn2 -- i_2_ph/RConn2
  Switch2/RConn2 -- i_3_ph/RConn2
  Switch3/RConn2 -- i_4_ph/RConn2
  Switch4/RConn2 -- i_5_ph/RConn2
  Switch5/RConn2 -- i_6_ph/RConn2
  Simulink-PS Converter/RConn1 -- Switch/RConn1 -- Switch1/RConn1 -- Switch2/RConn1 -- Switch3/RConn1 -- Switch4/RConn1 -- Switch5/RConn1

== system uz_mpc_6ph/inverter_machine/DC_link ==
  Capacitor : fl_lib/Electrical/Electrical Elements/Capacitor  c=C_dc_link uF  r=1e-6 Ohm  g=0 1/Ohm  i_specify=off  i_priority=None  i=0 A  i_nominal_specify=off  i_nominal_value=1  i_nominal_unit=A  v_specify=off  v_priority=None  v=0 V  v_nominal_specify=off  v_nominal_value=1  v_nominal_unit=V  vc_specify=off  vc_priority=High  vc=0 V  vc_nominal_specify=off  vc_nominal_value=1  vc_nominal_unit=V
  PS-Simulink Converter : nesl_utility/PS-Simulink Converter  PhysicalDomain=network_engine_domain  SubClassName=ps_output  LeftPortType=input  RightPortType=output  PseudoPeriodic=off  Frequencies=[]  VectorFormat=1-D array  Unit=1  AffineConversion=off
  Voltage Sensor : fl_lib/Electrical/Electrical Sensors/Voltage Sensor
  U_dc_link+_in : PMIOPort  Side=Left
  U_dc_link-_in : PMIOPort  Port=2  Side=Left
  U_dc_link+_out : PMIOPort  Port=3  Side=Right
  U_dc_link-_out : PMIOPort  Port=4  Side=Right
  u_dc_link_measured : Outport  VectorParamsAs1DForOutWhenUnconnected=off
  wires:
  PS-Simulink Converter/1 -> u_dc_link_measured/1
  connections:
  U_dc_link+_in/RConn1 -- Voltage Sensor/LConn1 -- U_dc_link+_out/RConn1 -- Capacitor/LConn1
  U_dc_link-_in/RConn1 -- Voltage Sensor/RConn2 -- U_dc_link-_out/RConn1 -- Capacitor/RConn1
  Voltage Sensor/RConn1 -- PS-Simulink Converter/LConn1

== system uz_mpc_6ph/inverter_machine/Power_Source ==
  Battery : batteryecm_lib/Battery  Vnom=v_dc V  prm_dir=1  R1_dis=2 Ohm  R1_ch=2 Ohm  R1=2 Ohm  prm_AH=1  AH=50 hr*A  V1=11.5 V  AH1=25 hr*A  prm_R2=1  R2=2000 Ohm  Tmeas=298.15 K  charge_measurement_port=simscape.enum.battery.enable.no  prm_dyn=1  Rp1=0.005 Ohm  tau1=30 s  Rp2=0.005 Ohm  tau2=30 s  Rp3=0.005 Ohm  tau3=30 s  Rp4=0.005 Ohm  tau4=30 s  Rp5=0.005 Ohm  tau5=30 s  prm_fade=1  N_fade=100  AH_fade=45 hr*A  R1_fade=2.02 Ohm  R1_ch_fade=2.02 Ohm  V1_fade=10.35 V  prm_age=1  prm_age_OCV=1  OCV_age=0.9  SOC_age=60  Tmeas_age=298.15 K  delta_time_age_vec=[0] d  temperature_age_vec=[273] K  OCV_scaling_age=2.2134e6  OCV_offset_age=1.632e6  temp_exp_age=0.515833569 V  t_exp_age=0.75  Vnom_T2=12 V  R1_T2=2.2 Ohm  R1_T2_dis=2.2 Ohm  R1_T2_ch=2.2 Ohm  V1_T2=11.4 V  R2_T2=2200 Ohm  Rp1_T2=0.005 Ohm  tau1_T2=30 s  Rp2_T2=0.005 Ohm  tau2_T2=30 s  Rp3_T2=0.005 Ohm  tau3_T2=30 s  Rp4_T2=0.005 Ohm  tau4_T2=30 s  Rp5_T2=0.005 Ohm  tau5_T2=30 s  Tmeas2=273.15 K  thermal_port=simscape.enum.thermaleffects.omit  thermal_mass=30000 J/K  i_specify=off  i_priority=None  i=0 A  i_nominal_specify=off  i_nominal_value=1  i_nominal_unit=A  v_specify=off  v_priority=None  v=0 V  v_nominal_specify=off  v_nominal_value=1  v_nominal_unit=V  charge_specify=off  charge_priority=High  charge=50 hr*A  charge_nominal_specify=off  charge_nominal_value=1  charge_nominal_unit=hr*A  num_cycles_specify=off  num_cycles_priority=High  num_cycles=0  num_cycles_nominal_specify=off  num_cycles_nominal_value=1  num_cycles_nominal_unit=1  temperature_specify=off  temperature_priority=High  temperature=298.15 K  temperature_nominal_specify=off  temperature_nominal_value=1  temperature_nominal_unit=K
  Controlled Voltage Source : fl_lib/Electrical/Electrical Sources/Controlled Voltage Source  Commented=on
  + : PMIOPort  Side=Right
  - : PMIOPort  Port=2  Side=Right
  ref_voltage : PMIOPort  Port=3  Side=Left
  connections:
  Battery/LConn1 -- +/RConn1
  Battery/RConn1 -- -/RConn1
  Controlled Voltage Source/RConn1 -- ref_voltage/RConn1

== system uz_mpc_6ph/mpc_enable/Subsystem2 ==
  Set : Inport
  Reset : Inport  Port=2
  Constant1 : Constant  Value=0  OutDataTypeStr=uint32  SampleTime=-1
  Data Type Conversion1 : DataTypeConversion  OutDataTypeStr=boolean  SaturateOnIntegerOverflow=off  RndMeth=Floor
  Data Type Conversion2 : DataTypeConversion  OutDataTypeStr=boolean  SaturateOnIntegerOverflow=off  RndMeth=Floor
  Logical Operator : Logic  Operator=NOT  AllPortsSameDT=off  OutDataTypeStr=boolean
  Logical Operator1 : Logic  AllPortsSameDT=off  OutDataTypeStr=boolean
  Logical Operator2 : Logic  Operator=OR  AllPortsSameDT=off  OutDataTypeStr=boolean
  Logical Operator3 : Logic  Operator=NOT  AllPortsSameDT=off  OutDataTypeStr=boolean
  Logical Operator4 : Logic  Operator=OR  AllPortsSameDT=off  OutDataTypeStr=boolean
  Logical Operator5 : Logic  AllPortsSameDT=off  OutDataTypeStr=boolean
  Switch1 : Switch  Criteria=u2 > Threshold  Threshold=1  SaturateOnIntegerOverflow=off  InputSameDT=off
  Unit Delay : UnitDelay  SampleTime=t_clock  HasFrameUpgradeWarning=on
  Q : Outport  VectorParamsAs1DForOutWhenUnconnected=off
  !Q : Outport  Port=2  VectorParamsAs1DForOutWhenUnconnected=off
  wires:
  Logical Operator/1 -> Logical Operator1/2, Logical Operator5/1
  Reset/1 -> Data Type Conversion2/1
  Constant1/1 -> Switch1/2
  Logical Operator4/1 -> Switch1/1
  Data Type Conversion1/1 -> Logical Operator2/1, Logical Operator4/1
  Switch1/1 -> Q/1, Unit Delay/1, Logical Operator3/1
  Logical Operator3/1 -> !Q/1
  Set/1 -> Data Type Conversion1/1
  Logical Operator2/1 -> Logical Operator1/1
  Unit Delay/1 -> Logical Operator2/2, Logical Operator5/2
  Logical Operator5/1 -> Logical Operator4/2
  Logical Operator1/1 -> Switch1/3
  Data Type Conversion2/1 -> Logical Operator/1

== system uz_mpc_6ph/uz_current_limit/RS_flipflop ==
  Set : Inport
  Reset : Inport  Port=2
  Constant1 : Constant  Value=0  OutDataTypeStr=uint32  SampleTime=-1
  Data Type Conversion1 : DataTypeConversion  OutDataTypeStr=boolean  SaturateOnIntegerOverflow=off  RndMeth=Floor
  Data Type Conversion2 : DataTypeConversion  OutDataTypeStr=boolean  SaturateOnIntegerOverflow=off  RndMeth=Floor
  Logical Operator : Logic  Operator=NOT  AllPortsSameDT=off  OutDataTypeStr=boolean
  Logical Operator1 : Logic  AllPortsSameDT=off  OutDataTypeStr=boolean
  Logical Operator2 : Logic  Operator=OR  AllPortsSameDT=off  OutDataTypeStr=boolean
  Logical Operator3 : Logic  Operator=NOT  AllPortsSameDT=off  OutDataTypeStr=boolean
  Logical Operator4 : Logic  Operator=OR  AllPortsSameDT=off  OutDataTypeStr=boolean
  Logical Operator5 : Logic  AllPortsSameDT=off  OutDataTypeStr=boolean
  Switch1 : Switch  Criteria=u2 > Threshold  Threshold=1  SaturateOnIntegerOverflow=off  InputSameDT=off
  Unit Delay : UnitDelay  SampleTime=t_clock  HasFrameUpgradeWarning=on
  Q : Outport  VectorParamsAs1DForOutWhenUnconnected=off
  !Q : Outport  Port=2  VectorParamsAs1DForOutWhenUnconnected=off
  wires:
  Logical Operator/1 -> Logical Operator1/2, Logical Operator5/1
  Reset/1 -> Data Type Conversion2/1
  Constant1/1 -> Switch1/2
  Logical Operator4/1 -> Switch1/1
  Data Type Conversion1/1 -> Logical Operator2/1, Logical Operator4/1
  Switch1/1 -> Q/1, Unit Delay/1, Logical Operator3/1
  Logical Operator3/1 -> !Q/1
  Set/1 -> Data Type Conversion1/1
  Logical Operator2/1 -> Logical Operator1/1
  Unit Delay/1 -> Logical Operator2/2, Logical Operator5/2
  Logical Operator5/1 -> Logical Operator4/2
  Logical Operator1/1 -> Switch1/3
  Data Type Conversion2/1 -> Logical Operator/1
